simulink model "c8mmimo"  (R2019b)
settings: Solver=VariableStepAuto  StartTime=0.0  StopTime=10.0  RelTol=1e-3  EnableMultiTasking=on
PreLoadFcn:
  | s=fotf('s'); g1=1/(1.35*s^1.2+2.3*s^0.9+1);
  | g2=2/(4.13*s^0.7+1); g4=-1/(3.8*s^0.8+1);
  | g3=1/(0.52*s^1.5+2.03*s^0.7+1); G=[g1,g2; g3,g4];
  | Kp=[-0.4596, -0.8881; -0.8503, 0.5262];
  | s=tf('s'); Kd=[-1/(2.5*s+1), 0; 0, -1/(s+1)];
  | s=fotf('s'); c1=10.7003+2.9743*s^-0.86736+15*s^0.7876;
  | c2=14.848+10.1421*s^-0.81932+14.6848*s^0.7355;
  | ww=[1e-5 1e5]; N=20;
  | u1=1; u2=0;
libraries: cstblocks x4
settings Model: Creator=Dingyu  LastModifiedBy=xuedi
settings DataIOCC: SaveFormat=Array  ReturnWorkspaceOutputs=off
settings OptimizationCC: LifeSpan=inf
settings DebuggingCC: SFUnexpectedBacktrackingDiag=warning  SFNoUnconditionalDefaultTransitionDiag=warning  SFExecutionAtInitializationDiag=none  ArithmeticOperatorsInVariantConditions=warning
settings SFSimCC: SimUseLocalCustomCode=off  CustomCodeUndefinedFunction=UseInterfaceOnly
settings RTWCC: RTWUseLocalCustomCode=off
settings CodeAppCC: StateflowObjectComments=on
settings GRTTargetCC: TargetLangStandard=C89/C90 (ANSI)
settings ConfigComp: CovMetricSettings=dw  CovSaveCumulativeToWorkspaceVar=on  CovSaveSingleToWorkspaceVar=on  CovExternalEMLEnable=off

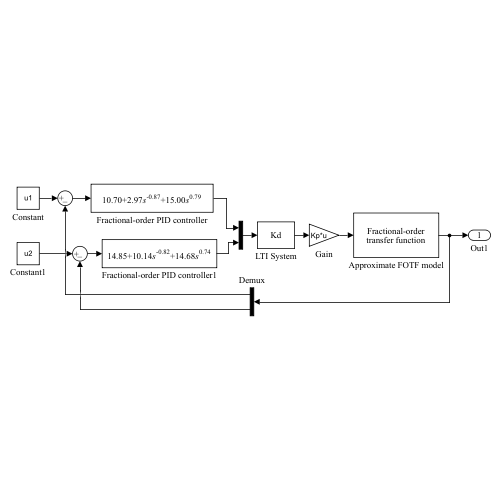
[thumbnail: Simulink's stored preview of the top-level diagram]
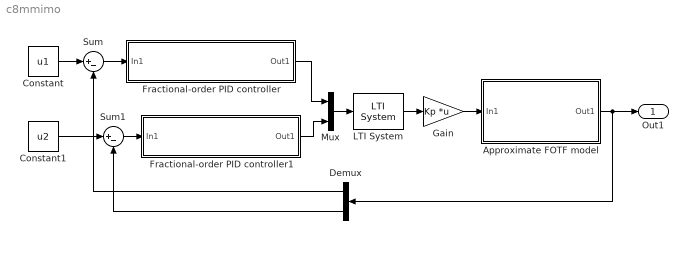
== system c8mmimo ==
  Approximate FOTF model : Subsystem  mask{na=G, a=[0.8 0.5 1], nb=0, b=1, ww=ww, N=N, kFilter=Oustaloup filter, T=0}
      mask prompts: na "Orders of the denominator"; a "Coefficients of the denominator"; nb "Orders of the numerator"; b "Coefficients of the numerator"; ww "Interested frequency range [wb wh]"; N "Filter order"; kFilter "Types of the filter"; T "Delay constant T"
      mask init:
      | if isa(na,'fotf'), G=na; 
      |    else
      |        if length(na)~=length(a)
      |           errordlg('Error','Mismatch on the denominator'), 
      |        end
      |        if length(b)~=length(nb)
      |           errordlg('Error','Mismatch on the numerator'), 
      |        end
      |        G=fotf(a,na,b,nb);
      |    end
      |    switch kFilter
      |       case 1, str='ousta_fod'; 
      |       case 2, str='new_fod'; case 3, str='matsude_fod';
      |    end
      |    wb=ww(1); wh=ww(2); G1=high_order(G,str,wb,wh,N); 
      |    G1.ioDelay=T;
      mask TypeOptions kFilter: Oustaloup filter | Modified Oustaloup filter
      mask Display: disp('Fractional-order\ntransfer function')
  Constant : Constant  Value=u1
  Constant1 : Constant  Value=u2
  Demux : Demux  Outputs=2
  Fractional-order PID controller : Subsystem  mask{Kp=c1, II=[0.4391 0.8647], DD=[1.1907 0.3844], N=N, ww=ww, kFilter=Oustaloup filter}
      mask prompts: Kp "Proportional Kp"; II "Integral [Ki lam]"; DD "Differentiation [Kd mu]"; N "Filter order"; ww "Interested frequency range [wb wh]"; kFilter "Types of the filter"
      mask init:
      | if isa(Kp,'fotf'), a=Kp;
      |    lam=a.den.na; mu=a.num.na; mu=mu(1)-lam; b=a.num.a; Kd=b(1); Kp=b(2); Ki=b(3);
      | else, II=[II 1]; DD=[DD 1]; Ki=II(1); lam=II(2); Kd=DD(1); mu=DD(2); end
      | s=fotf('s'); a=Kp+Ki/s^lam+Kd*s^mu/(0.001*s+1);
      | Gc=high_order(a,'ousta_fod',ww(1),ww(2),N);
      | if abs(Ki)>0, sI=[sprintf('%.2f',Ki),'{\its}^{' sprintf('%.2f',-lam), '}']; end
      | if abs(Kd)>0, sD=[sprintf('%.2f',Kd),'{\its}^{' sprintf('%.2f',mu), '}']; end
      | str=sprintf('%.2f',Kp);
      | if abs(Ki)>0, if sI(1)~='-', sI=['+' sI]; end, str=[str,sI]; end
      | if abs(Kd)>0, if sD(1)~='-', sD=['+' sD]; end, str=[str,sD]; end
      mask TypeOptions kFilter: Oustaloup filter | Modified Oustaloup filter
      mask Display: disp(str,'texmode','on')
  Fractional-order PID controller1 : Subsystem  mask{Kp=c2, II=[0.4391 0.8647], DD=[1.1907 0.3844], N=N, ww=ww, kFilter=Oustaloup filter}
      mask prompts: Kp "Proportional Kp"; II "Integral [Ki lam]"; DD "Differentiation [Kd mu]"; N "Filter order"; ww "Interested frequency range [wb wh]"; kFilter "Types of the filter"
      mask init: same as c8mmimo/Fractional-order PID controller
      mask TypeOptions kFilter: Oustaloup filter | Modified Oustaloup filter
      mask Display: disp(str,'texmode','on')
  Gain : Gain  Gain=Kp  Multiplication=Matrix(K*u)
  LTI System : cstblocks/LTI System  sys=Kd  IC=[]
  Mux : Mux  Inputs=2
  Sum : Sum  Inputs=|+-
  Sum1 : Sum  Inputs=|+-
  Out1 : Outport
  wires:
  Mux/1 -> LTI System/1
  LTI System/1 -> Gain/1
  Constant/1 -> Sum/1
  Sum/1 -> Fractional-order PID controller/1(In1)
  Sum1/1 -> Fractional-order PID controller1/1(In1)
  Constant1/1 -> Sum1/1
  Gain/1 -> Approximate FOTF model/1(In1)
  Demux/2 -> Sum1/2
  Demux/1 -> Sum/2
  Approximate FOTF model/1(Out1) -> Out1/1, Demux/1
  Fractional-order PID controller/1(Out1) -> Mux/1
  Fractional-order PID controller1/1(Out1) -> Mux/2

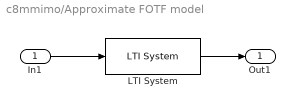
== system c8mmimo/Approximate FOTF model ==
  In1 : Inport
  LTI System : cstblocks/LTI System  sys=G1  IC=[]
  Out1 : Outport
  wires:
  LTI System/1 -> Out1/1
  In1/1 -> LTI System/1

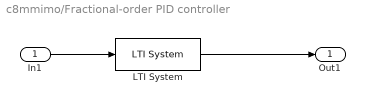
== system c8mmimo/Fractional-order PID controller ==
  In1 : Inport
  LTI System : cstblocks/LTI System  sys=Gc  IC=[]
  Out1 : Outport
  wires:
  In1/1 -> LTI System/1
  LTI System/1 -> Out1/1

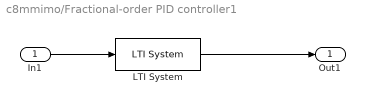
== system c8mmimo/Fractional-order PID controller1 ==
  In1 : Inport
  LTI System : cstblocks/LTI System  sys=Gc  IC=[]
  Out1 : Outport
  wires:
  LTI System/1 -> Out1/1
  In1/1 -> LTI System/1
